simulink model "clicktrasposta"  (R2024a)
settings: Solver=VariableStepAuto  StartTime=0.0  StopTime=100  RelTol=1e-3
undefined symbols (not defined in the file or in its folder): DiscIntNeverNeededParam
settings Model: Creator=paola  LastModifiedBy=UTENTE
settings RTWCC: GPUComputeCapability=3.5

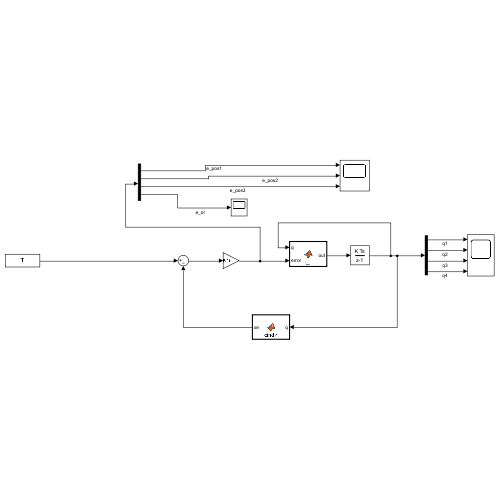
[thumbnail: Simulink's stored preview of the top-level diagram]
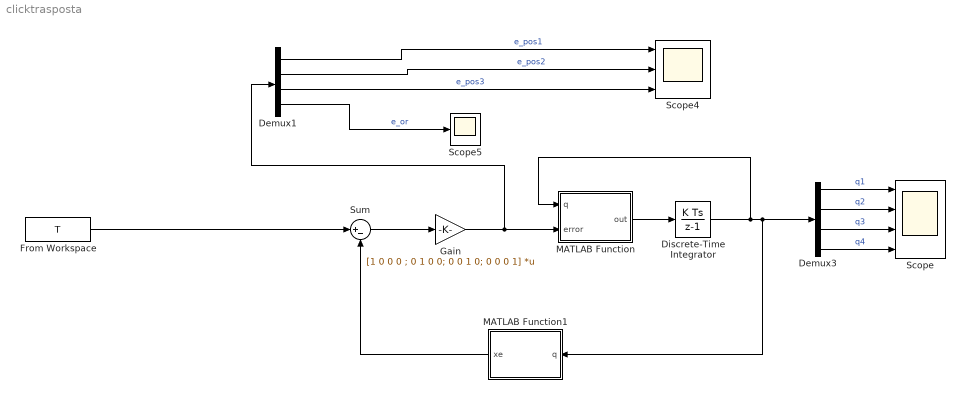
== system clicktrasposta ==
  Demux1 : Demux
  Demux3 : Demux
  Discrete-Time Integrator : DiscreteIntegrator  InitialCondition=[pi/6 pi/4 pi/5 0.5]'  SampleTime=0.001  ICPrevOutput=DiscIntNeverNeededParam  ICPrevScaledInput=DiscIntNeverNeededParam
  From Workspace : FromWorkspace  VariableName=T
  Gain : Gain  Gain=[1 0 0 0 ; 0 1 0 0; 0 0 1 0; 0 0 0 1]  Multiplication=Matrix(K*u)
  MATLAB Function : MATLAB Function  TreatAsAtomicUnit=on
  MATLAB Function1 : MATLAB Function  TreatAsAtomicUnit=on
  Scope : Scope  NumInputPorts=4
  Scope4 : Scope  NumInputPorts=3
  Scope5 : Scope
  Sum : Sum  Inputs=|+-
  wires:
  Sum/1 -> Gain/1
  Gain/1 -> Demux1/1, MATLAB Function/2(error)
  MATLAB Function1/1(xe) -> Sum/2
  MATLAB Function/1(out) -> Discrete-Time Integrator/1
  Discrete-Time Integrator/1 -> MATLAB Function/1(q), MATLAB Function1/1(q), Demux3/1
  Demux1/1 -> Scope4/1  "e_pos1"
  Demux3/1 -> Scope/1  "q1"
  Demux3/2 -> Scope/2  "q2"
  Demux3/3 -> Scope/3  "q3"
  Demux3/4 -> Scope/4  "q4"
  From Workspace/1 -> Sum/1
  Demux1/2 -> Scope4/2  "e_pos2"
  Demux1/3 -> Scope4/3  "e_pos3"
  Demux1/4 -> Scope5/1  "e_or"

== matlab function clicktrasposta/MATLAB Function ==
  data: q input; out output; error input
function out= i_j(q,error)
J=[-0.5*sin(q(1))-0.5*sin(q(1)+q(2)) -0.5*sin(q(1)+q(2)) 0 0;
    0.5*cos(q(1))+0.5*cos(q(1)+q(2)) 0.5*cos(q(1)+q(2)) 0 0;
    0 0 -1 0;
    1 1 0 -1];
J_t=(J');
%  trans_Jacobian=J_t;
out = J_t * error;
end

== matlab function clicktrasposta/MATLAB Function1 ==
  data: q input; xe output
function xe= cindir(q)
x_e=[0.5*cos(q(1))+0.5*cos(q(1)+q(2));
    0.5*sin(q(1))+0.5*sin(q(1)+q(2));
        1-q(3);
        q(1)+q(2)-q(4)];
xe=x_e;
end
